simulink model "sim_dist_att_obs_paper"  (R2020a)
settings: Solver=ode4  StartTime=0.0  StopTime=30.0  FixedStep=0.01  RelTol=1e-3
values from neighbouring files (symbols this model uses):
  beta_Phi_1 = pp0 * cal_frac_squ( 3, p_p0_plus_1, q_p0_plus_1 )                          * cal_frac_squ( eps_s_bar / pi, p_p0_min_2, q_p0_min_2 )                          / ( 2 * ( 2 * pp0 - 1 ) * tanh( gamma0 * ( eps_s_bar / pi ) / 2 ) )                          - ( cal_frac_squ( 3, p_p0_plus_1, q_p0_plus_1 ) * gamma0 / ( 4 * ( 2 * pp0 -1 ) ) )                          * cal_frac_squ( eps_s_bar / pi, p_p0_min_ ...(+136 chars)    [draw_compare_dist_att_obs.m]
  beta_Phi_2 = ( 1 - pp0 ) * cal_frac_squ( 3, p_p0_plus_1, q_p0_plus_1 )                          / ( 2 * ( 1 - 2 * pp0 ) * cal_frac_squ( eps_s_bar / pi, p_p0_0, q_p0_0 ) * tanh( gamma0 * ( eps_s_bar / pi ) / 2 ) )                          - ( cal_frac_squ( 3, p_p0_plus_1, q_p0_plus_1 ) * gamma0 / ( 4 * ( 1 - 2 * pp0 ) ) )                          * cal_frac_squ( eps_s_bar / pi, p_1_min_p0, q_1_min_p0 )          ...(+112 chars)    [draw_compare_dist_att_obs.m]
  c1_diff_sigma_bar_w = diag([12; 12; 12])    [draw_compare_dist_att_obs.m]
  c1_diff_ui = diag([25; 30; 20])    [draw_compare_dist_att_obs.m]
  c2_diff_sigma_bar_w = diag([12; 12; 12])    [draw_compare_dist_att_obs.m]
  c2_diff_ui = diag([50; 50; 10])    [draw_compare_dist_att_obs.m]
  c3_diff_sigma_bar_w = diag([15; 15; 15])    [draw_compare_dist_att_obs.m]
  c3_diff_ui = diag([15; 15; 10])    [draw_compare_dist_att_obs.m]
  c_w_1 = diag( [20; 15; 15] )    [draw_compare_dist_att_obs.m]
  c_w_2 = diag( [20; 15; 15] )    [draw_compare_dist_att_obs.m]
  c_w_3 = diag( [2; 2; 2] )    [draw_compare_dist_att_obs.m]
  cS0 = diag( [4.5; 4.5; 4.5] )    [draw_compare_dist_att_obs.m]
  dw_aa_t = 0.2 * ones(3, 5) + ( 1.0 - 0.2 ) * rand(3, 5)    [draw_compare_dist_att_obs.m]
  dw_ff_t = [ 0.4 * ones(1, 5) + ( 1.0 - 0.4 ) * rand(1, 5);                      0.4 * ones(1, 5) + ( 1.0 - 0.4 ) * rand(1, 5);                      0.2 * ones(1, 5) + ( 0.6 - 0.2 ) * rand(1, 5) ]    [draw_compare_dist_att_obs.m]
  dw_phi_t = ( - pi / 2 ) * ones(3, 5) + ( pi / 2 - ( - pi / 2 ) ) * rand(3, 5)    [draw_compare_dist_att_obs.m]
  dwci_init = zeros(3,5)    [draw_compare_dist_att_obs.m]
  eps_s_bar_div_pi = eps_s_bar / pi    (= 0.03)    [draw_compare_dist_att_obs.m]
  gamma0 = 20    [draw_compare_dist_att_obs.m]
  h1w = diag([20.0; 20.0; 20.0])    [draw_compare_dist_att_obs.m]
  h2w = diag([30.0; 35.0; 35.0])    [draw_compare_dist_att_obs.m]
  h3w = diag([30.0; 25.0; 30.0])    [draw_compare_dist_att_obs.m]
  Ji = zeros(3,3,NF)    [draw_compare_dist_att_obs.m]
  k_J_0 = diag( [1; 1; 1] )    [draw_compare_dist_att_obs.m]
  Lamd_diff_sigma_bar_w = 0.8    [draw_compare_dist_att_obs.m]
  Lamd_diff_ui = 0.8    [draw_compare_dist_att_obs.m]
  mu_c_theta = 100    [draw_compare_dist_att_obs.m]
  mu_d_w = 100    [draw_compare_dist_att_obs.m]
  pos0 = zeros(3, 1)    [draw_compare_dist_att_obs.m]
  pp0 = 8 / 11    (= 0.727272727273)    [draw_compare_dist_att_obs.m]
  PZ0 = P0(3)    [draw_compare_dist_att_obs.m]
  PZ1 = 10    [draw_compare_dist_att_obs.m]
  Qci_init = repmat([1;0;0;0],1,NF)    [draw_compare_dist_att_obs.m]
  R0 = 4    [draw_compare_dist_att_obs.m]
  R1 = 8    [draw_compare_dist_att_obs.m]
  Rci_init = zeros(3,3,NF)    [draw_compare_dist_att_obs.m]
  Ri_init = zeros(3,3,NF)    [draw_compare_dist_att_obs.m]
  Rx2 = 10    [draw_compare_dist_att_obs.m]
  Ry2 = 6    [draw_compare_dist_att_obs.m]
  Rz2 = 4    [draw_compare_dist_att_obs.m]
  T0 = 0    [draw_compare_dist_att_obs.m]
  T1 = tseq1    (= 10)    [draw_compare_dist_att_obs.m]
  T2 = tseq1 + tseq12 + tseq2    (= 30)    [draw_compare_dist_att_obs.m]
  thr_p_plus_1 = cal_frac_squ( 3, p_p0_plus_1, q_p0_plus_1 )    [draw_compare_dist_att_obs.m]
  ui_init = zeros(3,NF)    [draw_compare_dist_att_obs.m]
  vel0 = zeros(3, 1)    [draw_compare_dist_att_obs.m]
  wci_init = zeros(3,5)    [draw_compare_dist_att_obs.m]
  zeta_diff_sigma_bar_w = 0.3    [draw_compare_dist_att_obs.m]
  zeta_diff_ui = 0.05    [draw_compare_dist_att_obs.m]
undefined symbols (not defined in the file or in its folder): cal_frac_squ, p_2_p0, p_alfaw1, p_alfaw2, p_beta_w_1, p_beta_w_2, p_p0_min_1, p_p0_plus_1, q_2_p0, q_alfaw1, q_alfaw2, q_beta_w_1, q_beta_w_2, q_p0_min_1, q_p0_plus_1, Qei_init, Qi_init, Rei_init, V_Phi_Rei_init, wei_init, wi_init
(part 5 of 5)

== matlab function sim_dist_att_obs_paper/cal Phi_bar_psi_e agent 4 ==
  data: pp0 input; Phi_bar_psi_e_node_4 output; beta_Phi_1 input; beta_Phi_2 input; thr_p_plus_1 input; gamma0 input; eps_s_bar_div_pi input; wei_vec input; S_bar_vec input; V_Phi_Rei_div_pi_vec input; V_Phi_Rei_squ_p_min_1_vec input; V_Phi_Rei_squ_p_plus_1_vec input; V_Phi_Rei_squ_2p_vec input
function Phi_bar_psi_e_node_4 = fcn(pp0, beta_Phi_1, beta_Phi_2, thr_p_plus_1, gamma0, ...
                                                                    eps_s_bar_div_pi, wei_vec, S_bar_vec, V_Phi_Rei_div_pi_vec, ...
                                                                    V_Phi_Rei_squ_p_min_1_vec, V_Phi_Rei_squ_p_plus_1_vec, V_Phi_Rei_squ_2p_vec)
%%%% 计算姿态误差项
iiuav = 4;
Phi_bar_psi_e_node_4 = zeros(3,1);
for kk = 1:3
    if S_bar_vec(kk, iiuav) == 0
        Phi_bar_psi_e_node_4(kk, 1) = thr_p_plus_1 * ( pp0 + 1 ) * V_Phi_Rei_div_pi_vec(kk, iiuav) ...
                                                                * V_Phi_Rei_squ_p_min_1_vec(kk, iiuav) * wei_vec(kk, iiuav) ...
                                                                / ( 2 * tanh( ( gamma0 / 2 ) * V_Phi_Rei_div_pi_vec(kk, iiuav) ) ) ...
                                                                + ( thr_p_plus_1 * gamma0 / 4 ) * V_Phi_Rei_squ_p_plus_1_vec(kk, iiuav) ...
                                                                * ( ( sech( ( gamma0 / 2 ) * V_Phi_Rei_div_pi_vec(kk, iiuav) ) ...
                                                                / tanh( ( gamma0 / 2 ) * V_Phi_Rei_div_pi_vec(kk, iiuav) ) ) ^ 2 ) * wei_vec(kk, iiuav);
    else
        if abs( V_Phi_Rei_div_pi_vec ) > eps_s_bar_div_pi
            Phi_bar_psi_e_node_4(kk, 1) = thr_p_plus_1 * ( pp0 + 1 ) * V_Phi_Rei_div_pi_vec(kk, iiuav) ...
                                                                    * V_Phi_Rei_squ_p_min_1_vec(kk, iiuav) * wei_vec(kk, iiuav) ...
                                                                    / ( 2 * tanh( ( gamma0 / 2 ) * V_Phi_Rei_div_pi_vec(kk, iiuav) ) ) ...
                                                                    + ( thr_p_plus_1 * gamma0 / 4 ) * V_Phi_Rei_squ_p_plus_1_vec(kk, iiuav) ...
                                                                    * ( ( sech( ( gamma0 / 2 ) * V_Phi_Rei_div_pi_vec(kk, iiuav) ) ...
                                                                    / tanh( ( gamma0 / 2 ) * V_Phi_Rei_div_pi_vec(kk, iiuav) ) ) ^ 2 ) * wei_vec(kk, iiuav);
        else
            Phi_bar_psi_e_node_4(kk, 1) = 2 * beta_Phi_1 * ( ( abs( V_Phi_Rei_div_pi_vec(kk, iiuav) ) ) ^ 2 ) * wei_vec(kk, iiuav) ...
                                                                    + ( 2 * pp0 + 1 ) * beta_Phi_2 * V_Phi_Rei_squ_2p_vec(kk, iiuav) * wei_vec(kk, iiuav);
        end
    end
end

== matlab function sim_dist_att_obs_paper/trans to column67 ==
  data: x input; y output
function y = fcn(x)
y = x(:);

== matlab function sim_dist_att_obs_paper/trans to column68 ==
  data: x input; y output
function y = fcn(x)
y = x(:);

== matlab function sim_dist_att_obs_paper/trans to column69 ==
  data: x input; y output
function y = fcn(x)
y = x(:);

== matlab function sim_dist_att_obs_paper/trans to column70 ==
  data: x input; y output
function y = fcn(x)
y = x(:);

== matlab function sim_dist_att_obs_paper/trans to column71 ==
  data: x input; y output
function y = fcn(x)
y = x(:);

== matlab function sim_dist_att_obs_paper/trans to column72 ==
  data: x input; y output
function y = fcn(x)
y = x(:);

== matlab function sim_dist_att_obs_paper/trans to column73 ==
  data: x input; y output
function y = fcn(x)
y = x(:);

== matlab function sim_dist_att_obs_paper/trans to column74 ==
  data: x input; y output
function y = fcn(x)
y = x(:);

== matlab function sim_dist_att_obs_paper/trans to column75 ==
  data: x input; y output
function y = fcn(x)
y = x(:);

== matlab function sim_dist_att_obs_paper/trans to column76 ==
  data: x input; y output
function y = fcn(x)
y = x(:);

== matlab function sim_dist_att_obs_paper/trans to column77 ==
  data: x input; y output
function y = fcn(x)
y = x(:);

== matlab function sim_dist_att_obs_paper/trans to column78 ==
  data: x input; y output
function y = fcn(x)
y = x(:);

== matlab function sim_dist_att_obs_paper/trans to column79 ==
  data: x input; y output
function y = fcn(x)
y = x(:);

== matlab function sim_dist_att_obs_paper/trans to column80 ==
  data: x input; y output
function y = fcn(x)
y = x(:);

== matlab function sim_dist_att_obs_paper/trans to column81 ==
  data: x input; y output
function y = fcn(x)
y = x(:);

== matlab function sim_dist_att_obs_paper/trans to column82 ==
  data: x input; y output
function y = fcn(x)
y = x(:);

== matlab function sim_dist_att_obs_paper/trans to column83 ==
  data: x input; y output
function y = fcn(x)
y = x(:);

== matlab function sim_dist_att_obs_paper/trans to column84 ==
  data: x input; y output
function y = fcn(x)
y = x(:);

== matlab function sim_dist_att_obs_paper/trans to column85 ==
  data: x input; y output
function y = fcn(x)
y = x(:);

== matlab function sim_dist_att_obs_paper/trans to column86 ==
  data: x input; y output
function y = fcn(x)
y = x(:);

== matlab function sim_dist_att_obs_paper/trans to column87 ==
  data: x input; y output
function y = fcn(x)
y = x(:);

== matlab function sim_dist_att_obs_paper/trans to column88 ==
  data: x input; y output
function y = fcn(x)
y = x(:);

== matlab function sim_dist_att_obs_paper/trans to column89 ==
  data: x input; y output
function y = fcn(x)
y = x(:);

== matlab function sim_dist_att_obs_paper/trans to column90 ==
  data: x input; y output
function y = fcn(x)
y = x(:);

== matlab function sim_dist_att_obs_paper/trans to column91 ==
  data: x input; y output
function y = fcn(x)
y = x(:);

== matlab function sim_dist_att_obs_paper/cal Phi_bar_psi_e agent 5 ==
  data: pp0 input; Phi_bar_psi_e_node_5 output; beta_Phi_1 input; beta_Phi_2 input; thr_p_plus_1 input; gamma0 input; eps_s_bar_div_pi input; wei_vec input; S_bar_vec input; V_Phi_Rei_div_pi_vec input; V_Phi_Rei_squ_p_min_1_vec input; V_Phi_Rei_squ_p_plus_1_vec input; V_Phi_Rei_squ_2p_vec input
function Phi_bar_psi_e_node_5 = fcn(pp0, beta_Phi_1, beta_Phi_2, thr_p_plus_1, gamma0, ...
                                                                    eps_s_bar_div_pi, wei_vec, S_bar_vec, V_Phi_Rei_div_pi_vec, ...
                                                                    V_Phi_Rei_squ_p_min_1_vec, V_Phi_Rei_squ_p_plus_1_vec, V_Phi_Rei_squ_2p_vec)
%%%% 计算姿态误差项
iiuav = 5;
Phi_bar_psi_e_node_5 = zeros(3,1);
for kk = 1:3
    if S_bar_vec(kk, iiuav) == 0
        Phi_bar_psi_e_node_5(kk, 1) = thr_p_plus_1 * ( pp0 + 1 ) * V_Phi_Rei_div_pi_vec(kk, iiuav) ...
                                                                * V_Phi_Rei_squ_p_min_1_vec(kk, iiuav) * wei_vec(kk, iiuav) ...
                                                                / ( 2 * tanh( ( gamma0 / 2 ) * V_Phi_Rei_div_pi_vec(kk, iiuav) ) ) ...
                                                                + ( thr_p_plus_1 * gamma0 / 4 ) * V_Phi_Rei_squ_p_plus_1_vec(kk, iiuav) ...
                                                                * ( ( sech( ( gamma0 / 2 ) * V_Phi_Rei_div_pi_vec(kk, iiuav) ) ...
                                                                / tanh( ( gamma0 / 2 ) * V_Phi_Rei_div_pi_vec(kk, iiuav) ) ) ^ 2 ) * wei_vec(kk, iiuav);
    else
        if abs( V_Phi_Rei_div_pi_vec ) > eps_s_bar_div_pi
            Phi_bar_psi_e_node_5(kk, 1) = thr_p_plus_1 * ( pp0 + 1 ) * V_Phi_Rei_div_pi_vec(kk, iiuav) ...
                                                                    * V_Phi_Rei_squ_p_min_1_vec(kk, iiuav) * wei_vec(kk, iiuav) ...
                                                                    / ( 2 * tanh( ( gamma0 / 2 ) * V_Phi_Rei_div_pi_vec(kk, iiuav) ) ) ...
                                                                    + ( thr_p_plus_1 * gamma0 / 4 ) * V_Phi_Rei_squ_p_plus_1_vec(kk, iiuav) ...
                                                                    * ( ( sech( ( gamma0 / 2 ) * V_Phi_Rei_div_pi_vec(kk, iiuav) ) ...
                                                                    / tanh( ( gamma0 / 2 ) * V_Phi_Rei_div_pi_vec(kk, iiuav) ) ) ^ 2 ) * wei_vec(kk, iiuav);
        else
            Phi_bar_psi_e_node_5(kk, 1) = 2 * beta_Phi_1 * ( ( abs( V_Phi_Rei_div_pi_vec(kk, iiuav) ) ) ^ 2 ) * wei_vec(kk, iiuav) ...
                                                                    + ( 2 * pp0 + 1 ) * beta_Phi_2 * V_Phi_Rei_squ_2p_vec(kk, iiuav) * wei_vec(kk, iiuav);
        end
    end
end

== matlab function sim_dist_att_obs_paper/trans to column92 ==
  data: x input; y output
function y = fcn(x)
y = x(:);

== matlab function sim_dist_att_obs_paper/trans to column93 ==
  data: x input; y output
function y = fcn(x)
y = x(:);

== matlab function sim_dist_att_obs_paper/trans to column94 ==
  data: x input; y output
function y = fcn(x)
y = x(:);

== matlab function sim_dist_att_obs_paper/trans to column95 ==
  data: x input; y output
function y = fcn(x)
y = x(:);

== matlab function sim_dist_att_obs_paper/trans to column96 ==
  data: x input; y output
function y = fcn(x)
y = x(:);

== matlab function sim_dist_att_obs_paper/trans to column97 ==
  data: x input; y output
function y = fcn(x)
y = x(:);

== matlab function sim_dist_att_obs_paper/trans to column98 ==
  data: x input; y output
function y = fcn(x)
y = x(:);

== matlab function sim_dist_att_obs_paper/trans to column99 ==
  data: x input; y output
function y = fcn(x)
y = x(:);

== matlab function sim_dist_att_obs_paper/wi dynam agent 1 ==
  data: Ji input; dwi_1 output; wi_vec input; taui_vec input; dw_vec input
function dwi_1 = fcn(Ji, wi_vec, taui_vec, dw_vec)
%%%% 更新姿态角速率微分方程
iiuav = 1;
dwi_1 = inv(Ji(:,:,iiuav)) * ( -cal_askew_mat(wi_vec(:,iiuav)) * Ji(:,:,iiuav) * wi_vec(:,iiuav) ... 
                                                + taui_vec(:,iiuav) + dw_vec(:,iiuav) );

end

== matlab function sim_dist_att_obs_paper/wi dynam agent 2 ==
  data: Ji input; dwi_2 output; wi_vec input; taui_vec input; dw_vec input
function dwi_2 = fcn(Ji, wi_vec, taui_vec, dw_vec)
%%%% 更新姿态角速率微分方程
iiuav = 2;
dwi_2 = inv(Ji(:,:,iiuav)) * ( -cal_askew_mat(wi_vec(:,iiuav)) * Ji(:,:,iiuav) * wi_vec(:,iiuav) ... 
                                                + taui_vec(:,iiuav) + dw_vec(:,iiuav) );

end

== matlab function sim_dist_att_obs_paper/wi dynam agent 3 ==
  data: Ji input; dwi_3 output; wi_vec input; taui_vec input; dw_vec input
function dwi_3 = fcn(Ji, wi_vec, taui_vec, dw_vec)
%%%% 更新姿态角速率微分方程
iiuav = 3;
dwi_3 = inv(Ji(:,:,iiuav)) * ( -cal_askew_mat(wi_vec(:,iiuav)) * Ji(:,:,iiuav) * wi_vec(:,iiuav) ...
                                                + taui_vec(:,iiuav) + dw_vec(:,iiuav) );

end

== matlab function sim_dist_att_obs_paper/wi dynam agent 4 ==
  data: Ji input; dwi_4 output; wi_vec input; taui_vec input; dw_vec input
function dwi_4 = fcn(Ji, wi_vec, taui_vec, dw_vec)
%%%% 更新姿态角速率微分方程
iiuav = 4;
dwi_4 = inv(Ji(:,:,iiuav)) * ( -cal_askew_mat(wi_vec(:,iiuav)) * Ji(:,:,iiuav) * wi_vec(:,iiuav) ...
                                                + taui_vec(:,iiuav) + dw_vec(:,iiuav) );

end

== matlab function sim_dist_att_obs_paper/wi dynam agent 5 ==
  data: Ji input; dwi_5 output; wi_vec input; taui_vec input; dw_vec input
function dwi_5 = fcn(Ji, wi_vec, taui_vec, dw_vec)
%%%% 更新姿态角速率微分方程
iiuav = 5;
dwi_5 = inv(Ji(:,:,iiuav)) * ( -cal_askew_mat(wi_vec(:,iiuav)) * Ji(:,:,iiuav) * wi_vec(:,iiuav) ...
                                                + taui_vec(:,iiuav) + dw_vec(:,iiuav) );

end

== matlab function sim_dist_att_obs_paper/combine norminal formation control input ==
  data: ui_1 input; ui_vec output; ui_2 input; ui_3 input; ui_4 input; ui_5 input
function ui_vec = fcn(ui_1, ui_2, ui_3, ui_4, ui_5)
%%%% 合并领导者编队跟踪误差结果
ui_vec = [ui_1(:), ui_2(:), ui_3(:), ui_4(:), ui_5(:)];

== matlab function sim_dist_att_obs_paper/control input generator agent 1 ==
  data: u0 input; ui output
function ui  = fcn(u0)
%%%% 给出领导者参考加速度控制输入
g0 = 9.80663;
e3 = [0;0;1];

ui = g0 * e3 + u0(:);

== matlab function sim_dist_att_obs_paper/control input generator agent 2 ==
  data: u0 input; ui output
function ui  = fcn(u0)
%%%% 给出领导者参考加速度控制输入
g0 = 9.80663;
e3 = [0;0;1];

ui = g0 * e3 + u0(:);

== matlab function sim_dist_att_obs_paper/control input generator agent 3 ==
  data: u0 input; ui output
function ui  = fcn(u0)
%%%% 给出领导者参考加速度控制输入
g0 = 9.80663;
e3 = [0;0;1];

ui = g0 * e3 + u0(:);

== matlab function sim_dist_att_obs_paper/control input generator agent 4 ==
  data: u0 input; ui output
function ui  = fcn(u0)
%%%% 给出领导者参考加速度控制输入
g0 = 9.80663;
e3 = [0;0;1];

ui = g0 * e3 + u0(:);

== matlab function sim_dist_att_obs_paper/control input generator agent 5 ==
  data: u0 input; ui output
function ui  = fcn(u0)
%%%% 给出领导者参考加速度控制输入
g0 = 9.80663;
e3 = [0;0;1];

ui = g0 * e3 + u0(:);

== matlab function sim_dist_att_obs_paper/cal Phi_psi_e agent 1 ==
  data: Phi_psi_e_node_1 output; beta_Phi_1 input; beta_Phi_2 input; gamma0 input; thr_p_plus_1 input; eps_s_bar_div_pi input; S_bar_vec input; V_Phi_Rei_div_pi_vec input; V_Phi_Rei_squ_p_plus_1_vec input; V_Phi_Rei_squ_2p_vec input
function Phi_psi_e_node_1 = fcn(beta_Phi_1, beta_Phi_2, gamma0, thr_p_plus_1, eps_s_bar_div_pi, ...
                                                            S_bar_vec, V_Phi_Rei_div_pi_vec, ...
                                                            V_Phi_Rei_squ_p_plus_1_vec, V_Phi_Rei_squ_2p_vec)
%%%% 计算姿态误差项
iiuav = 1;
Phi_psi_e_node_1 = zeros(3,1);
for kk = 1:3
    if S_bar_vec(kk, iiuav) == 0
        Phi_psi_e_node_1(kk, 1) = ( thr_p_plus_1 * pi * V_Phi_Rei_squ_p_plus_1_vec(kk,iiuav) ) ...
                                                        / ( 2 * tanh( ( gamma0 / 2 ) * V_Phi_Rei_div_pi_vec(kk,iiuav) ) );
    else
        if abs( V_Phi_Rei_div_pi_vec ) > eps_s_bar_div_pi
            Phi_psi_e_node_1(kk, 1) = ( thr_p_plus_1 * pi * V_Phi_Rei_squ_p_plus_1_vec(kk,iiuav) ) ...
                                                            / ( 2 * tanh( ( gamma0 / 2 ) * V_Phi_Rei_div_pi_vec(kk,iiuav) ) );
        else
            Phi_psi_e_node_1(kk, 1) = V_Phi_Rei_div_pi_vec(kk, iiuav) * pi * ...
                                                            ( beta_Phi_1 * ( abs( V_Phi_Rei_div_pi_vec(kk, iiuav) ) ^ 2 ) ...
                                                            + beta_Phi_2 * V_Phi_Rei_squ_2p_vec(kk, iiuav) );
        end
    end
end

== matlab function sim_dist_att_obs_paper/cal Phi_psi_e agent 2 ==
  data: Phi_psi_e_node_2 output; beta_Phi_1 input; beta_Phi_2 input; gamma0 input; thr_p_plus_1 input; eps_s_bar_div_pi input; S_bar_vec input; V_Phi_Rei_div_pi_vec input; V_Phi_Rei_squ_p_plus_1_vec input; V_Phi_Rei_squ_2p_vec input
function Phi_psi_e_node_2 = fcn(beta_Phi_1, beta_Phi_2, gamma0, thr_p_plus_1, eps_s_bar_div_pi, ...
                                                            S_bar_vec, V_Phi_Rei_div_pi_vec, ...
                                                            V_Phi_Rei_squ_p_plus_1_vec, V_Phi_Rei_squ_2p_vec)
%%%% 计算姿态误差项
iiuav = 2;
Phi_psi_e_node_2 = zeros(3,1);
for kk = 1:3
    if S_bar_vec(kk, iiuav) == 0
        Phi_psi_e_node_2(kk, 1) = ( thr_p_plus_1 * pi * V_Phi_Rei_squ_p_plus_1_vec(kk,iiuav) ) ...
                                                        / ( 2 * tanh( ( gamma0 / 2 ) * V_Phi_Rei_div_pi_vec(kk,iiuav) ) );
    else
        if abs( V_Phi_Rei_div_pi_vec ) > eps_s_bar_div_pi
            Phi_psi_e_node_2(kk, 1) = ( thr_p_plus_1 * pi * V_Phi_Rei_squ_p_plus_1_vec(kk,iiuav) ) ...
                                                            / ( 2 * tanh( ( gamma0 / 2 ) * V_Phi_Rei_div_pi_vec(kk,iiuav) ) );
        else
            Phi_psi_e_node_2(kk, 1) = V_Phi_Rei_div_pi_vec(kk, iiuav) * pi * ...
                                                            ( beta_Phi_1 * ( abs( V_Phi_Rei_div_pi_vec(kk, iiuav) ) ^ 2 ) ...
                                                            + beta_Phi_2 * V_Phi_Rei_squ_2p_vec(kk, iiuav) );
        end
    end
end

== matlab function sim_dist_att_obs_paper/cal Phi_psi_e agent 3 ==
  data: Phi_psi_e_node_3 output; beta_Phi_1 input; beta_Phi_2 input; gamma0 input; thr_p_plus_1 input; eps_s_bar_div_pi input; S_bar_vec input; V_Phi_Rei_div_pi_vec input; V_Phi_Rei_squ_p_plus_1_vec input; V_Phi_Rei_squ_2p_vec input
function Phi_psi_e_node_3 = fcn(beta_Phi_1, beta_Phi_2, gamma0, thr_p_plus_1, eps_s_bar_div_pi, ...
                                                            S_bar_vec, V_Phi_Rei_div_pi_vec, ...
                                                            V_Phi_Rei_squ_p_plus_1_vec, V_Phi_Rei_squ_2p_vec)
%%%% 计算姿态误差项
iiuav = 3;
Phi_psi_e_node_3 = zeros(3,1);
for kk = 1:3
    if S_bar_vec(kk, iiuav) == 0
        Phi_psi_e_node_3(kk, 1) = ( thr_p_plus_1 * pi * V_Phi_Rei_squ_p_plus_1_vec(kk,iiuav) ) ...
                                                        / ( 2 * tanh( ( gamma0 / 2 ) * V_Phi_Rei_div_pi_vec(kk,iiuav) ) );
    else
        if abs( V_Phi_Rei_div_pi_vec ) > eps_s_bar_div_pi
            Phi_psi_e_node_3(kk, 1) = ( thr_p_plus_1 * pi * V_Phi_Rei_squ_p_plus_1_vec(kk,iiuav) ) ...
                                                            / ( 2 * tanh( ( gamma0 / 2 ) * V_Phi_Rei_div_pi_vec(kk,iiuav) ) );
        else
            Phi_psi_e_node_3(kk, 1) = V_Phi_Rei_div_pi_vec(kk, iiuav) * pi * ...
                                                            ( beta_Phi_1 * ( abs( V_Phi_Rei_div_pi_vec(kk, iiuav) ) ^ 2 ) ...
                                                            + beta_Phi_2 * V_Phi_Rei_squ_2p_vec(kk, iiuav) );
        end
    end
end

== matlab function sim_dist_att_obs_paper/cal Phi_psi_e agent 4 ==
  data: Phi_psi_e_node_4 output; beta_Phi_1 input; beta_Phi_2 input; gamma0 input; thr_p_plus_1 input; eps_s_bar_div_pi input; S_bar_vec input; V_Phi_Rei_div_pi_vec input; V_Phi_Rei_squ_p_plus_1_vec input; V_Phi_Rei_squ_2p_vec input
function Phi_psi_e_node_4 = fcn(beta_Phi_1, beta_Phi_2, gamma0, thr_p_plus_1, eps_s_bar_div_pi, ...
                                                            S_bar_vec, V_Phi_Rei_div_pi_vec, ...
                                                            V_Phi_Rei_squ_p_plus_1_vec, V_Phi_Rei_squ_2p_vec)
%%%% 计算姿态误差项
iiuav = 4;
Phi_psi_e_node_4 = zeros(3,1);
for kk = 1:3
    if S_bar_vec(kk, iiuav) == 0
        Phi_psi_e_node_4(kk, 1) = ( thr_p_plus_1 * pi * V_Phi_Rei_squ_p_plus_1_vec(kk,iiuav) ) ...
                                                        / ( 2 * tanh( ( gamma0 / 2 ) * V_Phi_Rei_div_pi_vec(kk,iiuav) ) );
    else
        if abs( V_Phi_Rei_div_pi_vec ) > eps_s_bar_div_pi
            Phi_psi_e_node_4(kk, 1) = ( thr_p_plus_1 * pi * V_Phi_Rei_squ_p_plus_1_vec(kk,iiuav) ) ...
                                                            / ( 2 * tanh( ( gamma0 / 2 ) * V_Phi_Rei_div_pi_vec(kk,iiuav) ) );
        else
            Phi_psi_e_node_4(kk, 1) = V_Phi_Rei_div_pi_vec(kk, iiuav) * pi * ...
                                                            ( beta_Phi_1 * ( abs( V_Phi_Rei_div_pi_vec(kk, iiuav) ) ^ 2 ) ...
                                                            + beta_Phi_2 * V_Phi_Rei_squ_2p_vec(kk, iiuav) );
        end
    end
end

== matlab function sim_dist_att_obs_paper/cal Phi_psi_e agent 5 ==
  data: Phi_psi_e_node_5 output; beta_Phi_1 input; beta_Phi_2 input; gamma0 input; thr_p_plus_1 input; eps_s_bar_div_pi input; S_bar_vec input; V_Phi_Rei_div_pi_vec input; V_Phi_Rei_squ_p_plus_1_vec input; V_Phi_Rei_squ_2p_vec input
function Phi_psi_e_node_5 = fcn(beta_Phi_1, beta_Phi_2, gamma0, thr_p_plus_1, eps_s_bar_div_pi, ...
                                                            S_bar_vec, V_Phi_Rei_div_pi_vec, ...
                                                            V_Phi_Rei_squ_p_plus_1_vec, V_Phi_Rei_squ_2p_vec)
%%%% 计算姿态误差项
iiuav = 5;
Phi_psi_e_node_5 = zeros(3,1);
for kk = 1:3
    if S_bar_vec(kk, iiuav) == 0
        Phi_psi_e_node_5(kk, 1) = ( thr_p_plus_1 * pi * V_Phi_Rei_squ_p_plus_1_vec(kk,iiuav) ) ...
                                                        / ( 2 * tanh( ( gamma0 / 2 ) * V_Phi_Rei_div_pi_vec(kk,iiuav) ) );
    else
        if abs( V_Phi_Rei_div_pi_vec ) > eps_s_bar_div_pi
            Phi_psi_e_node_5(kk, 1) = ( thr_p_plus_1 * pi * V_Phi_Rei_squ_p_plus_1_vec(kk,iiuav) ) ...
                                                            / ( 2 * tanh( ( gamma0 / 2 ) * V_Phi_Rei_div_pi_vec(kk,iiuav) ) );
        else
            Phi_psi_e_node_5(kk, 1) = V_Phi_Rei_div_pi_vec(kk, iiuav) * pi * ...
                                                            ( beta_Phi_1 * ( abs( V_Phi_Rei_div_pi_vec(kk, iiuav) ) ^ 2 ) ...
                                                            + beta_Phi_2 * V_Phi_Rei_squ_2p_vec(kk, iiuav) );
        end
    end
end

== matlab function sim_dist_att_obs_paper/cal Qci agent 1 ==
  data: Qi_vec input; Qci_1 output; Qei_vec input
function Qci_1 = fcn(Qi_vec, Qei_vec)
%%%% 更新期望指令四元数
iiuav = 1;

sigma1 = Qi_vec(1,iiuav);
q1 = Qi_vec(2:4,iiuav);
sigma2 = Qei_vec(1,iiuav);
q2 = -Qei_vec(2:4,iiuav);

sigma = sigma1*sigma2 - (q1')*q2;
q = sigma1*q2 + sigma2*q1 + cal_askew_mat(q1)*q2;
Qci_1 = [sigma; q];

end

== matlab function sim_dist_att_obs_paper/cal Qci agent 2 ==
  data: Qi_vec input; Qci_2 output; Qei_vec input
function Qci_2 = fcn(Qi_vec, Qei_vec)
%%%% 更新期望指令四元数
iiuav = 2;
sigma1 = Qi_vec(1,iiuav);
q1 = Qi_vec(2:4,iiuav);
sigma2 = Qei_vec(1,iiuav);
q2 = -Qei_vec(2:4,iiuav);

sigma = sigma1*sigma2 - (q1')*q2;
q = sigma1*q2 + sigma2*q1 + cal_askew_mat(q1)*q2;
Qci_2 = [sigma; q];

end

== matlab function sim_dist_att_obs_paper/cal Qci agent 3 ==
  data: Qi_vec input; Qci_3 output; Qei_vec input
function Qci_3 = fcn(Qi_vec, Qei_vec)
%%%% 更新期望指令四元数
iiuav = 3;
sigma1 = Qi_vec(1,iiuav);
q1 = Qi_vec(2:4,iiuav);
sigma2 = Qei_vec(1,iiuav);
q2 = -Qei_vec(2:4,iiuav);

sigma = sigma1*sigma2 - (q1')*q2;
q = sigma1*q2 + sigma2*q1 + cal_askew_mat(q1)*q2;
Qci_3 = [sigma; q];

end

== matlab function sim_dist_att_obs_paper/cal Qci agent 4 ==
  data: Qi_vec input; Qci_4 output; Qei_vec input
function Qci_4 = fcn(Qi_vec, Qei_vec)
%%%% 更新期望指令四元数
iiuav = 4;
sigma1 = Qi_vec(1,iiuav);
q1 = Qi_vec(2:4,iiuav);
sigma2 = Qei_vec(1,iiuav);
q2 = -Qei_vec(2:4,iiuav);

sigma = sigma1*sigma2 - (q1')*q2;
q = sigma1*q2 + sigma2*q1 + cal_askew_mat(q1)*q2;
Qci_4 = [sigma; q];

end

== matlab function sim_dist_att_obs_paper/cal Qci agent 5 ==
  data: Qi_vec input; Qci_5 output; Qei_vec input
function Qci_5 = fcn(Qi_vec, Qei_vec)
%%%% 更新期望指令四元数
iiuav = 5;
sigma1 = Qi_vec(1,iiuav);
q1 = Qi_vec(2:4,iiuav);
sigma2 = Qei_vec(1,iiuav);
q2 = -Qei_vec(2:4,iiuav);

sigma = sigma1*sigma2 - (q1')*q2;
q = sigma1*q2 + sigma2*q1 + cal_askew_mat(q1)*q2;
Qci_5 = [sigma; q];

end

== matlab function sim_dist_att_obs_paper/cal Rci agent 1 ==
  data: Rci_1 output; Qci input
function Rci_1 = fcn(Qci)
%%%% 使用罗德里格公式由四元数Qci求解Rci
thetaci_tmp = Qci(1,1);
qci_tmp = Qci(2:4,1);
Rci_1 = ((thetaci_tmp^2) - (qci_tmp')*qci_tmp) * eye(3,3) ...
                + 2 * qci_tmp * (qci_tmp') ...
                - 2 * thetaci_tmp * cal_askew_mat(qci_tmp);

end

== matlab function sim_dist_att_obs_paper/cal Rci agent 2 ==
  data: Rci_2 output; Qci input
function Rci_2 = fcn(Qci)
%%%% 使用罗德里格公式由四元数Qci求解Rci

thetaci_tmp = Qci(1,1);
qci_tmp = Qci(2:4,1);
Rci_2 = ((thetaci_tmp^2) - (qci_tmp')*qci_tmp) * eye(3,3) ...
                + 2 * qci_tmp * (qci_tmp') ...
                - 2 * thetaci_tmp * cal_askew_mat(qci_tmp);

end

== matlab function sim_dist_att_obs_paper/cal Rci agent 3 ==
  data: Rci_3 output; Qci input
function Rci_3 = fcn(Qci)
%%%% 使用罗德里格公式由四元数Qci求解Rci
thetaci_tmp = Qci(1,1);
qci_tmp = Qci(2:4,1);
Rci_3 = ((thetaci_tmp^2) - (qci_tmp')*qci_tmp) * eye(3,3) ...
                + 2 * qci_tmp * (qci_tmp') ...
                - 2 * thetaci_tmp * cal_askew_mat(qci_tmp);

end

== matlab function sim_dist_att_obs_paper/cal Rci agent 4 ==
  data: Rci_4 output; Qci input
function Rci_4 = fcn(Qci)
%%%% 使用罗德里格公式由四元数Qci求解Rci
thetaci_tmp = Qci(1,1);
qci_tmp = Qci(2:4,1);
Rci_4 = ((thetaci_tmp^2) - (qci_tmp')*qci_tmp) * eye(3,3) ...
                + 2 * qci_tmp * (qci_tmp') ...
                - 2 * thetaci_tmp * cal_askew_mat(qci_tmp);

end

== matlab function sim_dist_att_obs_paper/cal Rci agent 5 ==
  data: Rci_5 output; Qci_vec input
function Rci_5 = fcn(Qci_vec)
%%%% 使用罗德里格公式由四元数Qci求解Rci
thetaci_tmp = Qci_vec(1,1);
qci_tmp = Qci_vec(2:4,1);
Rci_5 = ((thetaci_tmp^2) - (qci_tmp')*qci_tmp) * eye(3,3) ...
                + 2 * qci_tmp * (qci_tmp') ...
                - 2 * thetaci_tmp * cal_askew_mat(qci_tmp);

end

== matlab function sim_dist_att_obs_paper/cal Rei agent 1 ==
  data: Rei_1 output; Qei_vec input
function Rei_1 = fcn(Qei_vec)
%%%% 使用罗德里格公式由四元数Qei求解Rei
iiuav = 1;
thetaei_tmp = Qei_vec(1,iiuav);
qei_tmp = Qei_vec(2:4,iiuav);
Rei_1 = ((thetaei_tmp^2) - (qei_tmp')*qei_tmp) * eye(3,3) ...
                + 2 * qei_tmp * (qei_tmp') ...
                - 2 * thetaei_tmp * cal_askew_mat(qei_tmp);

end

== matlab function sim_dist_att_obs_paper/cal Rei agent 2 ==
  data: Rei_2 output; Qei_vec input
function Rei_2 = fcn(Qei_vec)
%%%% 使用罗德里格公式由四元数Qei求解Rei
iiuav = 2;
thetaei_tmp = Qei_vec(1,iiuav);
qei_tmp = Qei_vec(2:4,iiuav);
Rei_2 = ((thetaei_tmp^2) - (qei_tmp')*qei_tmp) * eye(3,3) ...
                + 2 * qei_tmp * (qei_tmp') ...
                - 2 * thetaei_tmp * cal_askew_mat(qei_tmp);

end

== matlab function sim_dist_att_obs_paper/cal Rei agent 3 ==
  data: Rei_3 output; Qei_vec input
function Rei_3 = fcn(Qei_vec)
%%%% 使用罗德里格公式由四元数Qei求解Rei
iiuav = 3;
thetaei_tmp = Qei_vec(1,iiuav);
qei_tmp = Qei_vec(2:4,iiuav);
Rei_3 = ((thetaei_tmp^2) - (qei_tmp')*qei_tmp) * eye(3,3) ...
                + 2 * qei_tmp * (qei_tmp') ...
                - 2 * thetaei_tmp * cal_askew_mat(qei_tmp);

end

== matlab function sim_dist_att_obs_paper/cal Rei agent 4 ==
  data: Rei_4 output; Qei_vec input
function Rei_4 = fcn(Qei_vec)
%%%% 使用罗德里格公式由四元数Qei求解Rei
iiuav = 4;
thetaei_tmp = Qei_vec(1,iiuav);
qei_tmp = Qei_vec(2:4,iiuav);
Rei_4 = ((thetaei_tmp^2) - (qei_tmp')*qei_tmp) * eye(3,3) ...
                + 2 * qei_tmp * (qei_tmp') ...
                - 2 * thetaei_tmp * cal_askew_mat(qei_tmp);

end

== matlab function sim_dist_att_obs_paper/cal Rei agent 5 ==
  data: Rei_5 output; Qei_vec input
function Rei_5 = fcn(Qei_vec)
%%%% 使用罗德里格公式由四元数Qei求解Rei
iiuav = 5;
thetaei_tmp = Qei_vec(1,iiuav);
qei_tmp = Qei_vec(2:4,iiuav);
Rei_5 = ((thetaei_tmp^2) - (qei_tmp')*qei_tmp) * eye(3,3) ...
                + 2 * qei_tmp * (qei_tmp') ...
                - 2 * thetaei_tmp * cal_askew_mat(qei_tmp);

end

== matlab function sim_dist_att_obs_paper/cal Ri agent 1 ==
  data: Ri_1 output; Qi_vec input
function Ri_1 = fcn(Qi_vec)
%%%% 使用罗德里格公式由四元数Qi求解Ri
iiuav = 1;
thetai_tmp = Qi_vec(1,iiuav);
qi_tmp = Qi_vec(2:4,iiuav);
Ri_1 = ((thetai_tmp^2) - (qi_tmp')*qi_tmp) * eye(3,3) ...
            + 2 * qi_tmp * (qi_tmp') ...
            - 2 * thetai_tmp * cal_askew_mat(qi_tmp);

end

== matlab function sim_dist_att_obs_paper/cal Ri agent 2 ==
  data: Ri_2 output; Qi_vec input
function Ri_2 = fcn(Qi_vec)
%%%% 使用罗德里格公式由四元数Qi求解Ri
iiuav = 2;
thetai_tmp = Qi_vec(1,iiuav);
qi_tmp = Qi_vec(2:4,iiuav);
Ri_2 = ((thetai_tmp^2) - (qi_tmp')*qi_tmp) * eye(3,3) ...
            + 2 * qi_tmp * (qi_tmp') ...
            - 2 * thetai_tmp * cal_askew_mat(qi_tmp);

end

== matlab function sim_dist_att_obs_paper/cal Ri agent 3 ==
  data: Ri_3 output; Qi_vec input
function Ri_3 = fcn(Qi_vec)
%%%% 使用罗德里格公式由四元数Qi求解Ri
iiuav = 3;
thetai_tmp = Qi_vec(1,iiuav);
qi_tmp = Qi_vec(2:4,iiuav);
Ri_3 = ((thetai_tmp^2) - (qi_tmp')*qi_tmp) * eye(3,3) ...
            + 2 * qi_tmp * (qi_tmp') ...
            - 2 * thetai_tmp * cal_askew_mat(qi_tmp);

end

== matlab function sim_dist_att_obs_paper/cal Ri agent 4 ==
  data: Ri_4 output; Qi_vec input
function Ri_4 = fcn(Qi_vec)
%%%% 使用罗德里格公式由四元数Qi求解Ri
iiuav = 4;
thetai_tmp = Qi_vec(1,iiuav);
qi_tmp = Qi_vec(2:4,iiuav);
Ri_4 = ((thetai_tmp^2) - (qi_tmp')*qi_tmp) * eye(3,3) ...
            + 2 * qi_tmp * (qi_tmp') ...
            - 2 * thetai_tmp * cal_askew_mat(qi_tmp);

end

== matlab function sim_dist_att_obs_paper/cal Ri agent 5 ==
  data: Ri_5 output; Qi_vec input
function Ri_5 = fcn(Qi_vec)
%%%% 使用罗德里格公式由四元数Qi求解Ri
iiuav = 5;
thetai_tmp = Qi_vec(1,iiuav);
qi_tmp = Qi_vec(2:4,iiuav);
Ri_5 = ((thetai_tmp^2) - (qi_tmp')*qi_tmp) * eye(3,3) ...
            + 2 * qi_tmp * (qi_tmp') ...
            - 2 * thetai_tmp * cal_askew_mat(qi_tmp);

end

== matlab function sim_dist_att_obs_paper/cal S_bar agent 1 ==
  data: cS0 input; gamma0 input; thr_p_plus_1 input; wei_vec input; S_bar_node_1 output; V_Phi_Rei_div_pi_vec input; V_Phi_Rei_squ_p_plus_1_vec input
function S_bar_node_1 = fcn(cS0, gamma0, thr_p_plus_1, wei_vec, ...
                                                        V_Phi_Rei_div_pi_vec, V_Phi_Rei_squ_p_plus_1_vec)
%%%% 计算辅助滑模面
iiuav = 1;
S_bar_node_1 = zeros(3,1);
for kk = 1:3
S_bar_node_1(kk,1) = wei_vec(kk,iiuav) + cS0(kk, kk) * ( thr_p_plus_1 * pi * V_Phi_Rei_squ_p_plus_1_vec(kk,iiuav) ) ...
                                        / ( 2 * tanh( ( gamma0 / 2 ) * V_Phi_Rei_div_pi_vec(kk,iiuav) ) );
end

== matlab function sim_dist_att_obs_paper/cal S_bar agent 2 ==
  data: cS0 input; gamma0 input; thr_p_plus_1 input; wei_vec input; S_bar_node_2 output; V_Phi_Rei_div_pi_vec input; V_Phi_Rei_squ_p_plus_1_vec input
function S_bar_node_2 = fcn(cS0, gamma0, thr_p_plus_1, wei_vec, ...
                                                        V_Phi_Rei_div_pi_vec, V_Phi_Rei_squ_p_plus_1_vec)
%%%% 计算辅助滑模面
iiuav = 2;
S_bar_node_2 = zeros(3,1);
for kk = 1:3
S_bar_node_2(kk,1) = wei_vec(kk,iiuav) + cS0(kk, kk) * ( thr_p_plus_1 * pi * V_Phi_Rei_squ_p_plus_1_vec(kk,iiuav) ) ...
                                        / ( 2 * tanh( ( gamma0 / 2 ) * V_Phi_Rei_div_pi_vec(kk,iiuav) ) );
end

== matlab function sim_dist_att_obs_paper/cal S_bar agent 3 ==
  data: cS0 input; gamma0 input; thr_p_plus_1 input; wei_vec input; S_bar_node_3 output; V_Phi_Rei_div_pi_vec input; V_Phi_Rei_squ_p_plus_1_vec input
function S_bar_node_3 = fcn(cS0, gamma0, thr_p_plus_1, wei_vec, ...
                                                        V_Phi_Rei_div_pi_vec, V_Phi_Rei_squ_p_plus_1_vec)
%%%% 计算辅助滑模面
iiuav = 3;
S_bar_node_3 = zeros(3,1);
for kk = 1:3
S_bar_node_3(kk,1) = wei_vec(kk,iiuav) + cS0(kk, kk) * ( thr_p_plus_1 * pi * V_Phi_Rei_squ_p_plus_1_vec(kk,iiuav) ) ...
                                        / ( 2 * tanh( ( gamma0 / 2 ) * V_Phi_Rei_div_pi_vec(kk,iiuav) ) );
end

== matlab function sim_dist_att_obs_paper/cal S_bar agent 4 ==
  data: cS0 input; gamma0 input; thr_p_plus_1 input; wei_vec input; S_bar_node_4 output; V_Phi_Rei_div_pi_vec input; V_Phi_Rei_squ_p_plus_1_vec input
function S_bar_node_4 = fcn(cS0, gamma0, thr_p_plus_1, wei_vec, ...
                                                        V_Phi_Rei_div_pi_vec, V_Phi_Rei_squ_p_plus_1_vec)
%%%% 计算辅助滑模面
iiuav = 4;
S_bar_node_4 = zeros(3,1);
for kk = 1:3
S_bar_node_4(kk,1) = wei_vec(kk,iiuav) + cS0(kk, kk) * ( thr_p_plus_1 * pi * V_Phi_Rei_squ_p_plus_1_vec(kk,iiuav) ) ...
                                        / ( 2 * tanh( ( gamma0 / 2 ) * V_Phi_Rei_div_pi_vec(kk,iiuav) ) );
end

== matlab function sim_dist_att_obs_paper/cal S_bar agent 5 ==
  data: cS0 input; gamma0 input; thr_p_plus_1 input; wei_vec input; S_bar_node_5 output; V_Phi_Rei_div_pi_vec input; V_Phi_Rei_squ_p_plus_1_vec input
function S_bar_node_5 = fcn(cS0, gamma0, thr_p_plus_1, wei_vec, ...
                                                        V_Phi_Rei_div_pi_vec, V_Phi_Rei_squ_p_plus_1_vec)
%%%% 计算辅助滑模面
iiuav = 5;
S_bar_node_5 = zeros(3,1);
for kk = 1:3
S_bar_node_5(kk,1) = wei_vec(kk,iiuav) + cS0(kk, kk) * ( thr_p_plus_1 * pi * V_Phi_Rei_squ_p_plus_1_vec(kk,iiuav) ) ...
                                        / ( 2 * tanh( ( gamma0 / 2 ) * V_Phi_Rei_div_pi_vec(kk,iiuav) ) );
end

== matlab function sim_dist_att_obs_paper/cal Si agent 1 ==
  data: cS0 input; wei_vec input; Phi_psi_e_vec input; Si_1 output
function Si_1 = fcn(cS0, wei_vec, Phi_psi_e_vec)
%%%% 计算滑模面
iiuav = 1;
Si_1 = zeros(3,1);
for kk = 1:3
    Si_1(kk, 1) = wei_vec(kk, iiuav) + cS0(kk, kk) * Phi_psi_e_vec(kk, iiuav);
end

== matlab function sim_dist_att_obs_paper/cal Si agent 2 ==
  data: cS0 input; wei_vec input; Phi_psi_e_vec input; Si_2 output
function Si_2 = fcn(cS0, wei_vec, Phi_psi_e_vec)
%%%% 计算滑模面
iiuav = 2;
Si_2 = zeros(3,1);
for kk = 1:3
    Si_2(kk, 1) = wei_vec(kk, iiuav) + cS0(kk, kk) * Phi_psi_e_vec(kk, iiuav);
end

== matlab function sim_dist_att_obs_paper/cal Si agent 3 ==
  data: cS0 input; wei_vec input; Phi_psi_e_vec input; Si_3 output
function Si_3 = fcn(cS0, wei_vec, Phi_psi_e_vec)
%%%% 计算滑模面
iiuav = 3;
Si_3 = zeros(3,1);
for kk = 1:3
    Si_3(kk, 1) = wei_vec(kk, iiuav) + cS0(kk, kk) * Phi_psi_e_vec(kk, iiuav);
end

== matlab function sim_dist_att_obs_paper/cal Si agent 4 ==
  data: cS0 input; wei_vec input; Phi_psi_e_vec input; Si_4 output
function Si_4 = fcn(cS0, wei_vec, Phi_psi_e_vec)
%%%% 计算滑模面
iiuav = 4;
Si_4 = zeros(3,1);
for kk = 1:3
    Si_4(kk, 1) = wei_vec(kk, iiuav) + cS0(kk, kk) * Phi_psi_e_vec(kk, iiuav);
end

== matlab function sim_dist_att_obs_paper/cal Si agent 5 ==
  data: cS0 input; wei_vec input; Phi_psi_e_vec input; Si_5 output
function Si_5 = fcn(cS0, wei_vec, Phi_psi_e_vec)
%%%% 计算滑模面
iiuav = 5;
Si_5 = zeros(3,1);
for kk = 1:3
    Si_5(kk, 1) = wei_vec(kk, iiuav) + cS0(kk, kk) * Phi_psi_e_vec(kk, iiuav);
end

== matlab function sim_dist_att_obs_paper/cal abs 61 ==
  data: x input; y output
function y = fcn(x)
y = abs(x(:));

== matlab function sim_dist_att_obs_paper/cal abs 62 ==
  data: x input; y output
function y = fcn(x)
y = abs(x(:));

== matlab function sim_dist_att_obs_paper/cal abs 63 ==
  data: x input; y output
function y = fcn(x)
y = abs(x(:));

== matlab function sim_dist_att_obs_paper/cal abs 64 ==
  data: x input; y output
function y = fcn(x)
y = abs(x(:));

== matlab function sim_dist_att_obs_paper/cal abs 65 ==
  data: x input; y output
function y = fcn(x)
y = abs(x(:));

== matlab function sim_dist_att_obs_paper/cal abs 66 ==
  data: x input; y output
function y = fcn(x)
y = abs(x(:));

== matlab function sim_dist_att_obs_paper/cal abs 67 ==
  data: x input; y output
function y = fcn(x)
y = abs(x(:));

== matlab function sim_dist_att_obs_paper/cal abs 68 ==
  data: x input; y output
function y = fcn(x)
y = abs(x(:));

== matlab function sim_dist_att_obs_paper/cal abs 69 ==
  data: x input; y output
function y = fcn(x)
y = abs(x(:));

== matlab function sim_dist_att_obs_paper/cal abs 70 ==
  data: x input; y output
function y = fcn(x)
y = abs(x(:));

== matlab function sim_dist_att_obs_paper/cal abs 71 ==
  data: x input; y output
function y = fcn(x)
y = abs(x(:));

== matlab function sim_dist_att_obs_paper/cal abs 72 ==
  data: x input; y output
function y = fcn(x)
y = abs(x(:));

== matlab function sim_dist_att_obs_paper/cal abs 73 ==
  data: x input; y output
function y = fcn(x)
y = abs(x(:));

== matlab function sim_dist_att_obs_paper/cal abs 74 ==
  data: x input; y output
function y = fcn(x)
y = abs(x(:));

== matlab function sim_dist_att_obs_paper/cal abs 75 ==
  data: x input; y output
function y = fcn(x)
y = abs(x(:));

== matlab function sim_dist_att_obs_paper/cal abs 76 ==
  data: x input; y output
function y = fcn(x)
y = abs(x(:));

== matlab function sim_dist_att_obs_paper/cal abs 77 ==
  data: x input; y output
function y = fcn(x)
y = abs(x(:));

== matlab function sim_dist_att_obs_paper/cal abs 78 ==
  data: x input; y output
function y = fcn(x)
y = abs(x(:));

== matlab function sim_dist_att_obs_paper/cal abs 79 ==
  data: x input; y output
function y = fcn(x)
y = abs(x(:));

== matlab function sim_dist_att_obs_paper/cal abs 80 ==
  data: x input; y output
function y = fcn(x)
y = abs(x(:));

== matlab function sim_dist_att_obs_paper/cal abs 81 ==
  data: x input; y output
function y = fcn(x)
y = abs(x(:));

== matlab function sim_dist_att_obs_paper/cal abs 82 ==
  data: x input; y output
function y = fcn(x)
y = abs(x(:));

== matlab function sim_dist_att_obs_paper/cal abs 83 ==
  data: x input; y output
function y = fcn(x)
y = abs(x(:));

== matlab function sim_dist_att_obs_paper/cal abs 84 ==
  data: x input; y output
function y = fcn(x)
y = abs(x(:));

== matlab function sim_dist_att_obs_paper/cal abs 85 ==
  data: x input; y output
function y = fcn(x)
y = abs(x(:));

== matlab function sim_dist_att_obs_paper/cal abs 86 ==
  data: x input; y output
function y = fcn(x)
y = abs(x(:));

== matlab function sim_dist_att_obs_paper/leader control input ==
  data: t input; u0 output; T1 input; T2 input; R0 input; R1 input; Rx2 input; Ry2 input; Rz2 input
function u0  = fcn(t, T1, T2, R0, R1, Rx2, Ry2, Rz2)
%%%% 给出领导者参考加速度控制输入
u0 = zeros(3, 1);

if t <= ( T1 + 1e-05 )
    u0(1, 1) = - ( 4 * pi * sin( ( 2 * pi * ( t - 0 ) ) / ( 0 - T1 ) ) * ( R0 - R1 ) ) / ( ( 0 - T1 ) ^ 2 ) ...
                        - ( 4 * ( pi ^ 2 ) * cos( ( 2 * pi * ( t - 0 ) ) / ( 0 - T1 ) ) ...
                        * ( R0 + ( ( R0 - R1 ) * ( t - 0 ) ) / ( 0 - T1 ) ) ) / ( ( 0 - T1 ) ^ 2 );
    u0(2, 1) = ( 4 * pi * cos( ( 2 * pi * ( t - 0 ) ) / ( 0 - T1 ) ) * ( R0 - R1 ) ) / ( ( 0 - T1 ) ^ 2 ) ...
                        - ( 4 * ( pi ^ 2 ) * sin( ( 2 * pi * ( t - 0 ) ) / ( 0 - T1 ) ) ...
                        * ( R0 + ( ( R0 - R1 ) * ( t - 0 ) ) / ( 0 - T1 ) ) ) / ( ( 0 - T1 ) ^ 2 );
    u0(3, 1) = 0;
else
    u0(1, 1) = ( 4 * Rx2 * ( pi ^ 2 ) * cos( ( 2 * pi * ( t - T1 ) ) / ( T1 - T2 ) ) ) / ( ( T1 - T2 ) ^ 2 );
    u0(2, 1) = - ( 16 * Ry2 * ( pi ^ 2 ) * sin( ( 4 * pi * ( t - T1 ) ) / ( T1 - T2 ) ) ) / ( ( T1 - T2 ) ^ 2 );
    u0(3, 1) = ( 16 * Rz2 * ( pi ^ 2 ) * sin( ( 4 * pi * ( t - T1 ) ) / ( T1 - T2 ) ) ) / ( ( T1 - T2 ) ^ 2 );
end

== matlab function sim_dist_att_obs_paper/cal abs 87 ==
  data: x input; y output
function y = fcn(x)
y = abs(x(:));

== matlab function sim_dist_att_obs_paper/cal abs 88 ==
  data: x input; y output
function y = fcn(x)
y = abs(x(:));

== matlab function sim_dist_att_obs_paper/cal abs 89 ==
  data: x input; y output
function y = fcn(x)
y = abs(x(:));

== matlab function sim_dist_att_obs_paper/cal abs 90 ==
  data: x input; y output
function y = fcn(x)
y = abs(x(:));

== matlab function sim_dist_att_obs_paper/cal abs 91 ==
  data: x input; y output
function y = fcn(x)
y = abs(x(:));

== matlab function sim_dist_att_obs_paper/cal abs 92 ==
  data: x input; y output
function y = fcn(x)
y = abs(x(:));

== matlab function sim_dist_att_obs_paper/cal abs 93 ==
  data: x input; y output
function y = fcn(x)
y = abs(x(:));

== matlab function sim_dist_att_obs_paper/cal abs 94 ==
  data: x input; y output
function y = fcn(x)
y = abs(x(:));

== matlab function sim_dist_att_obs_paper/cal abs 95 ==
  data: x input; y output
function y = fcn(x)
y = abs(x(:));

== matlab function sim_dist_att_obs_paper/cal combine sigma_bar_w_tilt ==
  data: sigma_bar_w_vec input; sigma_bar_w_hat_vec input; sigma_bar_w_tilt_vec output
function sigma_bar_w_tilt_vec = fcn(sigma_bar_w_vec, sigma_bar_w_hat_vec)
%%%% 计算虚拟速度观测误差sigma_bar_w_tilt
sigma_bar_w_tilt_vec = zeros(3,5);
for iiuav = 1:5
    sigma_bar_w_tilt_vec(:,iiuav) = sigma_bar_w_vec(:,iiuav) - sigma_bar_w_hat_vec(:,iiuav);
end

== matlab function sim_dist_att_obs_paper/cal d_sigma_w agent 1 ==
  data: h3w input; d_sigma_w_1 output; Ji input; wi_vec input; taui_vec input; sigma_w_bar_vec input
function d_sigma_w_1 = fcn(h3w, Ji, wi_vec, taui_vec, sigma_w_bar_vec)
%%%% 计算辅助姿态角速率导数
iiuav = 1;
d_sigma_w_1 = inv(Ji(:,:,iiuav)) * ( -cal_askew_mat(wi_vec(:,iiuav)) * Ji(:,:,iiuav) * wi_vec(:,iiuav) ...
                            + taui_vec(:,iiuav) + h3w * sigma_w_bar_vec(:,iiuav) );

== matlab function sim_dist_att_obs_paper/cal d_sigma_w agent 2 ==
  data: h3w input; d_sigma_w_2 output; Ji input; wi_vec input; taui_vec input; sigma_w_bar_vec input
function d_sigma_w_2 = fcn(h3w, Ji, wi_vec, taui_vec, sigma_w_bar_vec)
%%%% 计算辅助姿态角速率导数
iiuav = 2;
d_sigma_w_2 = inv(Ji(:,:,iiuav)) * ( -cal_askew_mat(wi_vec(:,iiuav)) * Ji(:,:,iiuav) * wi_vec(:,iiuav) ...
                            + taui_vec(:,iiuav) + h3w * sigma_w_bar_vec(:,iiuav) );

== matlab function sim_dist_att_obs_paper/cal d_sigma_w agent 3 ==
  data: h3w input; d_sigma_w_3 output; Ji input; wi_vec input; taui_vec input; sigma_w_bar_vec input
function d_sigma_w_3 = fcn(h3w, Ji, wi_vec, taui_vec, sigma_w_bar_vec)
%%%% 计算辅助姿态角速率导数
iiuav = 3;
d_sigma_w_3 = inv(Ji(:,:,iiuav)) * ( -cal_askew_mat(wi_vec(:,iiuav)) * Ji(:,:,iiuav) * wi_vec(:,iiuav) ...
                            + taui_vec(:,iiuav) + h3w * sigma_w_bar_vec(:,iiuav) );

== matlab function sim_dist_att_obs_paper/cal d_sigma_w agent 4 ==
  data: h3w input; d_sigma_w_4 output; Ji input; wi_vec input; taui_vec input; sigma_w_bar_vec input
function d_sigma_w_4 = fcn(h3w, Ji, wi_vec, taui_vec, sigma_w_bar_vec)
%%%% 计算辅助姿态角速率导数
iiuav = 4;
d_sigma_w_4 = inv(Ji(:,:,iiuav)) * ( -cal_askew_mat(wi_vec(:,iiuav)) * Ji(:,:,iiuav) * wi_vec(:,iiuav) ...
                            + taui_vec(:,iiuav) + h3w * sigma_w_bar_vec(:,iiuav) );

== matlab function sim_dist_att_obs_paper/cal d_sigma_w agent 5 ==
  data: h3w input; d_sigma_w_5 output; Ji input; wi_vec input; taui_vec input; sigma_w_bar_vec input
function d_sigma_w_5 = fcn(h3w, Ji, wi_vec, taui_vec, sigma_w_bar_vec)
%%%% 计算辅助姿态角速率导数
iiuav = 5;
d_sigma_w_5 = inv(Ji(:,:,iiuav)) * ( -cal_askew_mat(wi_vec(:,iiuav)) * Ji(:,:,iiuav) * wi_vec(:,iiuav) ...
                            + taui_vec(:,iiuav) + h3w * sigma_w_bar_vec(:,iiuav) );

== matlab function sim_dist_att_obs_paper/cal d_theta_hat ==
  data: c1 input; d_ui_hat output; d_dui_hat output; d_d2ui_hat output; c2 input; c3 input; chi_t input; ui_sig_1 input; ui_sig_2 input; ui_sig_3 input; ui_sig_4 input; ui_sig_5 input; ui_sig_6 input; dui_hat input; d2ui_hat input
function [d_ui_hat, d_dui_hat, d_d2ui_hat] = fcn(c1, c2, c3, chi_t, ui_sig_1, ui_sig_2, ui_sig_3, ...
                                                                                        ui_sig_4, ui_sig_5, ui_sig_6, dui_hat, d2ui_hat)
d_d2ui_hat = -chi_t .* c1 * ui_sig_1(:) - (1 - chi_t) .* c1 * ui_sig_2(:);
d_dui_hat = -chi_t .* c2 * ui_sig_3(:) - (1 - chi_t) .* c2 * ui_sig_4(:) + d2ui_hat(:);
d_ui_hat = -chi_t .* c3 * ui_sig_5(:) - (1 - chi_t) .* c3 * ui_sig_6(:) + dui_hat(:);
